simulink model "SysGen_Radar"  (R2017b)
settings: Solver=VariableStepAuto  StartTime=0.0  StopTime=inf  RelTol=1e-3
libraries: xbsIndex_r4 x21
settings Model: Creator=Norbi  LastModifiedBy=Norbi

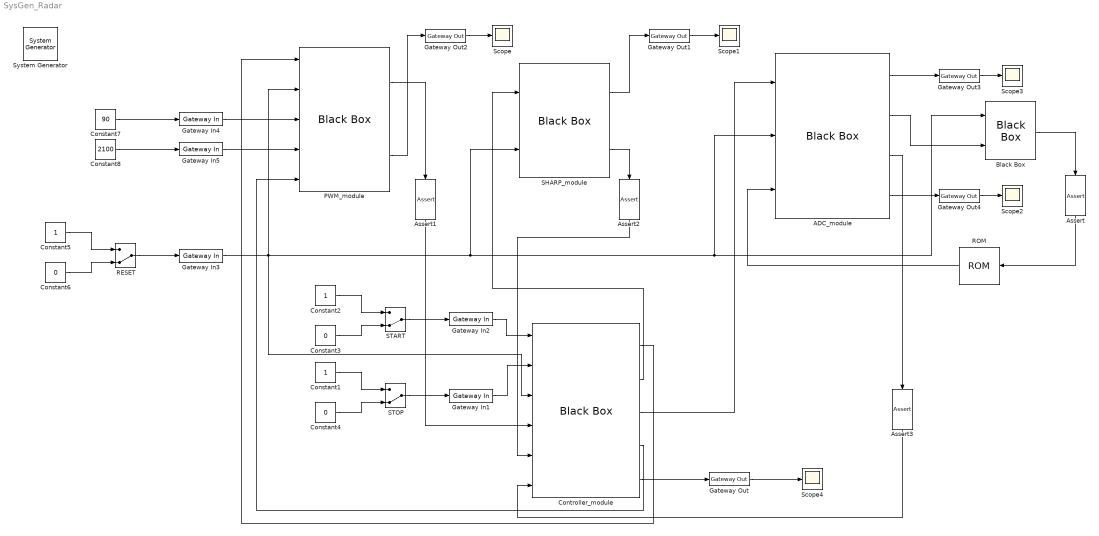
== system SysGen_Radar ==
  " System Generator" : xbsIndex_r4/ System Generator  Tag=genX  xilinxfamily=zynq  part=xc7z010  speed=-1  package=clg400  synthesis_tool=Vivado  clock_wrapper=Clock Enables  directory=./netlist  proj_type=Vivado  Synth_file=Vivado Synthesis Defaults  Impl_file=Vivado Implementation Defaults  testbench=off  simulink_period=1  sysclk_period=10  dcm_input_clock_period=10  incr_netlist=off  trim_vbits=Everywhere in SubSystem  dbl_ovrd=According to Block Masks  core_generation=According to Block Masks  run_coregen=off  deprecated_control=off  eval_field=0  block_type=sysgen
  ADC_module : xbsIndex_r4/Black Box  init_code=ADC_module_config  sim_method=ISE Simulator  verbose=off  block_type=blackbox2
  Assert{,1..3} (4 alike) : xbsIndex_r4/Assert  assert_type=off  type_source=Explicitly  gui_display_data_type=Fixed-point  arith_type="Signed  (2's comp)"  n_bits=16  bin_pt=14  preci_type=Single  exp_width=8  frac_width=24  assert_rate=on  rate_source=Explicitly  period=1  output_port=on  block_type=assert
  Black Box : xbsIndex_r4/Black Box  init_code=Counter_module_config  sim_method=ISE Simulator  verbose=off  block_type=blackbox2
  Constant1 : Constant  OutDataTypeStr=fixdt(1,16,0)
  Constant2 : Constant  OutDataTypeStr=fixdt(1,16,0)
  Constant3 : Constant  Value=0  OutDataTypeStr=fixdt(1,16,0)
  Constant4 : Constant  Value=0  OutDataTypeStr=fixdt(1,16,0)
  Constant5 : Constant  OutDataTypeStr=fixdt(1,16,0)
  Constant6 : Constant  Value=0  OutDataTypeStr=fixdt(1,16,0)
  Constant7 : Constant  Value=90  OutDataTypeStr=fixdt(1,16,0)
  Constant8 : Constant  Value=2100  OutDataTypeStr=fixdt(1,16,0)
  Controller_module : xbsIndex_r4/Black Box  init_code=Controller_module_config  sim_method=ISE Simulator  verbose=off  block_type=blackbox2
  Gateway In1 : xbsIndex_r4/Gateway In  gui_display_data_type=Fixed-point  arith_type="Signed  (2's comp)"  n_bits=1  bin_pt=0  preci_type=Single  exp_width=8  frac_width=24  rows=1  columns=1  quantization="Round  (unbiased: +/- Inf)"  overflow=Saturate  period=1  UseAsADC=off  ADCChannel='1'  interface=None  automatic_assignment=on  address_offset=hex2dec('00')  intf_name=''  intf_description=''  default_value=0  timing_constraint=None  locs_specified=off  LOCs={}  io_standard={}  inherit_from_input=off  hdl_port=on  dbl_ovrd=off  block_type=gatewayin
  Gateway In2 : xbsIndex_r4/Gateway In  gui_display_data_type=Fixed-point  arith_type="Signed  (2's comp)"  n_bits=1  bin_pt=0  preci_type=Single  exp_width=8  frac_width=24  rows=1  columns=1  quantization="Round  (unbiased: +/- Inf)"  overflow=Saturate  period=1  UseAsADC=off  ADCChannel='1'  interface=None  automatic_assignment=on  address_offset=hex2dec('00')  intf_name=''  intf_description=''  default_value=0  timing_constraint=None  locs_specified=off  LOCs={}  io_standard={}  inherit_from_input=off  hdl_port=on  dbl_ovrd=off  block_type=gatewayin
  Gateway In3 : xbsIndex_r4/Gateway In  gui_display_data_type=Fixed-point  arith_type="Signed  (2's comp)"  n_bits=1  bin_pt=0  preci_type=Single  exp_width=8  frac_width=24  rows=1  columns=1  quantization="Round  (unbiased: +/- Inf)"  overflow=Saturate  period=1  UseAsADC=off  ADCChannel='1'  interface=None  automatic_assignment=on  address_offset=hex2dec('00')  intf_name=''  intf_description=''  default_value=0  timing_constraint=None  locs_specified=off  LOCs={}  io_standard={}  inherit_from_input=off  hdl_port=on  dbl_ovrd=off  block_type=gatewayin
  Gateway In4 : xbsIndex_r4/Gateway In  gui_display_data_type=Fixed-point  arith_type="Signed  (2's comp)"  n_bits=11  bin_pt=0  preci_type=Single  exp_width=8  frac_width=24  rows=1  columns=1  quantization="Round  (unbiased: +/- Inf)"  overflow=Saturate  period=1  UseAsADC=off  ADCChannel='1'  interface=None  automatic_assignment=on  address_offset=hex2dec('00')  intf_name=''  intf_description=''  default_value=0  timing_constraint=None  locs_specified=off  LOCs={}  io_standard={}  inherit_from_input=off  hdl_port=on  dbl_ovrd=off  block_type=gatewayin
  Gateway In5 : xbsIndex_r4/Gateway In  gui_display_data_type=Fixed-point  arith_type="Signed  (2's comp)"  n_bits=11  bin_pt=0  preci_type=Single  exp_width=8  frac_width=24  rows=1  columns=1  quantization="Round  (unbiased: +/- Inf)"  overflow=Saturate  period=1  UseAsADC=off  ADCChannel='1'  interface=None  automatic_assignment=on  address_offset=hex2dec('00')  intf_name=''  intf_description=''  default_value=0  timing_constraint=None  locs_specified=off  LOCs={}  io_standard={}  inherit_from_input=off  hdl_port=on  dbl_ovrd=off  block_type=gatewayin
  Gateway Out{,1..4} (5 alike) : xbsIndex_r4/Gateway Out  inherit_from_input=off  hdl_port=on  rows=1  columns=1  UseAsDAC=off  DACChannel='1'  interface=None  automatic_assignment=on  address_offset=hex2dec('00')  intf_name=''  intf_description=''  timing_constraint=None  locs_specified=off  LOCs={}  io_standard={}  block_type=gatewayout
  PWM_module : xbsIndex_r4/Black Box  init_code=PWM_module_config  sim_method=ISE Simulator  verbose=off  block_type=blackbox2
  RESET : ManualSwitch  CurrentSetting=0
  ROM : xbsIndex_r4/ROM  depth=16  initVector=[0,0,0,1,1,0,0,0,0,0,0,0,1,0,1]  distributed_mem=Block RAM  rst=off  init_reg=0  en=off  latency=1  gui_display_data_type=Fixed-point  arith_type="Signed  (2's comp)"  n_bits=1  bin_pt=0  preci_type=Single  exp_width=8  frac_width=24  optimize=Area  use_rpm=on  dbl_ovrd=off  block_type=sprom
  SHARP_module : xbsIndex_r4/Black Box  init_code=SHARP_module_config  sim_method=ISE Simulator  verbose=off  block_type=blackbox2
  START : ManualSwitch  CurrentSetting=0
  STOP : ManualSwitch  CurrentSetting=0
  Scope{,1..4} (5 alike) : Scope
  wires:
  START/1 -> Gateway In2/1
  Constant3/1 -> START/2
  Constant2/1 -> START/1
  Constant1/1 -> STOP/1
  STOP/1 -> Gateway In1/1
  Constant4/1 -> STOP/2
  Gateway In2/1 -> Controller_module/1
  Gateway In1/1 -> Controller_module/2
  Constant5/1 -> RESET/1
  RESET/1 -> Gateway In3/1
  Constant6/1 -> RESET/2
  Gateway In3/1 -> Black Box/1, ADC_module/2, SHARP_module/2, Controller_module/3, PWM_module/2
  Controller_module/1 -> PWM_module/1
  Controller_module/2 -> SHARP_module/1
  Controller_module/3 -> ADC_module/1
  Controller_module/4 -> PWM_module/5
  PWM_module/1 -> Assert1/1
  SHARP_module/2 -> Assert2/1
  ADC_module/3 -> Assert3/1
  ROM/1 -> ADC_module/3
  Gateway In4/1 -> PWM_module/3
  Constant7/1 -> Gateway In4/1
  Constant8/1 -> Gateway In5/1
  Gateway In5/1 -> PWM_module/4
  ADC_module/2 -> Black Box/2
  Black Box/1 -> Assert/1
  Assert/1 -> ROM/1
  Assert1/1 -> Controller_module/4
  Assert2/1 -> Controller_module/5
  Assert3/1 -> Controller_module/6
  Gateway Out/1 -> Scope4/1
  Controller_module/5 -> Gateway Out/1
  Gateway Out1/1 -> Scope1/1
  SHARP_module/1 -> Gateway Out1/1
  Gateway Out2/1 -> Scope/1
  PWM_module/2 -> Gateway Out2/1
  Gateway Out3/1 -> Scope3/1
  ADC_module/1 -> Gateway Out3/1
  Gateway Out4/1 -> Scope2/1
  ADC_module/4 -> Gateway Out4/1
